simulink model "rigLoggerMultipacketRigH"  (R2012b)
settings: Solver=FixedStepDiscrete  StartTime=0.0  StopTime=10.0  FixedStep=0.001  RelTol=1e-3
values from neighbouring files (symbols this model uses):
  modelConstants = modelDefinedConstants()    [multipacketTestStart.m]
undefined symbols (not defined in the file or in its folder): macaddr
libraries: simulink x42, xpcethernetlib x29, xpcnetworkbufferlib x15, xpcutilitieslib x14, dspswit3 x14, dspmtrx3 x14, Lib_FileLoggerMultipacket x1
(part 1 of 6)
settings Model: BufferReuse=off  Creator=gilja  LastModifiedBy=NPTL
settings SolverCC: EnableConcurrentExecution=on  ConcurrentTasks=on
settings DataIOCC: SaveOutput=off  SignalLogging=off  SaveTime=off
settings OptimizationCC: InlineParams=on  InlineInvariantSignals=on  OptimizeBlockIOStorage=off  BufferReuse=off  ExpressionFolding=off  LocalBlockOutputs=off  SimCompilerOptimization=On
settings HardwareCC: ProdIntDivRoundTo=Zero  ProdEndianess=LittleEndian  ProdHWDeviceType=Generic->32-bit x86 compatible
settings ModelReferenceCC: ModelReferenceNumInstancesAllowed=Single  ModelReferenceMinAlgLoopOccurrences=on
settings RTWCC: SystemTargetFile=xpctarget.tlc  TemplateMakefile=xpc_default_tmf  Description=xPC Target  ProcessScript=xpctarget_make_rtw_hook  RTWCompilerOptimization=On
settings CodeAppCC: MaxIdLength=62
settings xpcTargetCC: TargetFcnLib=ansi_tfl_table_tmw.mat  CodeReplacementLibrary=XPC_BLAS  ParMdlRefBuildCompliant=on  ConcurrentExecutionCompliant=on  CombineSignalStateStructs=off  GRTInterface=on  RL32LogTETModifier=off  xPCTaskExecutionProfile=off  xPCRL32EventNumber=5000  xPCisDownloadable=off  xPCLoadParamSetFile=off  xPCConcurrentTasks=off  xPCEnableSFAnimation=off

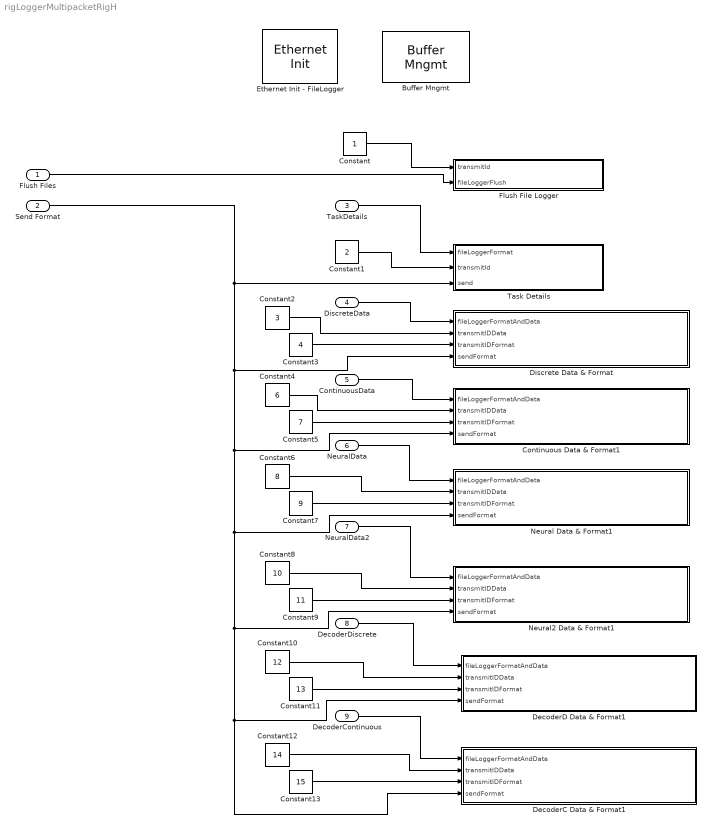
== system rigLoggerMultipacketRigH ==
  Flush Files : Inport  OutDataTypeStr=boolean
  Send Format : Inport  Port=2  OutDataTypeStr=boolean
  TaskDetails : Inport  Port=3  OutDataTypeStr=Bus: fileLoggerFormat
  DiscreteData : Inport  Port=4  OutDataTypeStr=Bus: fileLoggerFormatAndData
  ContinuousData : Inport  Port=5  OutDataTypeStr=Bus: fileLoggerFormatAndData
  NeuralData : Inport  Port=6  OutDataTypeStr=Bus: fileLoggerFormatAndData
  NeuralData2 : Inport  Port=7  OutDataTypeStr=Bus: fileLoggerFormatAndData
  DecoderDiscrete : Inport  Port=8  OutDataTypeStr=Bus: fileLoggerFormatAndData
  DecoderContinuous : Inport  Port=9  OutDataTypeStr=Bus: fileLoggerFormatAndData
  "Buffer Mngmt " : xpcnetworkbufferlib/Buffer Mngmt   Priority=-1  SampleTime=-1  PoolSizes=[8196 512 4096 65535]  ShowTune=on
  Constant : Constant  OutDataTypeStr=uint8
  Constant1 : Constant  Value=2  OutDataTypeStr=uint8
  Constant10 : Constant  Value=12  OutDataTypeStr=uint8
  Constant11 : Constant  Value=13  OutDataTypeStr=uint8
  Constant12 : Constant  Value=14  OutDataTypeStr=uint8
  Constant13 : Constant  Value=15  OutDataTypeStr=uint8
  Constant2 : Constant  Value=3  OutDataTypeStr=uint8
  Constant3 : Constant  Value=4  OutDataTypeStr=uint8
  Constant4 : Constant  Value=6  OutDataTypeStr=uint8
  Constant5 : Constant  Value=7  OutDataTypeStr=uint8
  Constant6 : Constant  Value=8  OutDataTypeStr=uint8
  Constant7 : Constant  Value=9  OutDataTypeStr=uint8
  Constant8 : Constant  Value=10  OutDataTypeStr=uint8
  Constant9 : Constant  Value=11  OutDataTypeStr=uint8
  Continuous Data & Format1 : Subsystem
  DecoderC Data & Format1 : Subsystem
  DecoderD Data & Format1 : Subsystem
  Discrete Data & Format : Subsystem
  Ethernet Init - FileLogger : xpcethernetlib/Ethernet Init   Priority=-1  ID=2  Driver=Intel Gigabit  Bus=6  Slot=0  SampleTime=-1  AddressSource=Specify  MAC=macaddr('00:00:00:00:00:00')  TxSA=off  RxPromiscuous=off  Multicast={}  RxBad=off  RxShort=off  MaxMTU=1518  TxThreshold=10  TxBuffers=128  RxBuffers=8  ShowTune=on  NumRxBlks=1
  Flush File Logger : Subsystem
  Neural Data & Format1 : Subsystem
  Neural2 Data & Format1 : Subsystem
  Task Details : Subsystem
  wires:
  Flush Files/1 -> Flush File Logger/2(fileLoggerFlush)
  TaskDetails/1 -> Task Details/1(fileLoggerFormat)
  ContinuousData/1 -> Continuous Data & Format1/1(fileLoggerFormatAndData)
  DiscreteData/1 -> Discrete Data & Format/1(fileLoggerFormatAndData)
  NeuralData/1 -> Neural Data & Format1/1(fileLoggerFormatAndData)
  DecoderDiscrete/1 -> DecoderD Data & Format1/1(fileLoggerFormatAndData)
  DecoderContinuous/1 -> DecoderC Data & Format1/1(fileLoggerFormatAndData)
  Send Format/1 -> Task Details/3(send), Discrete Data & Format/4(sendFormat), Continuous Data & Format1/4(sendFormat), Neural Data & Format1/4(sendFormat), Neural2 Data & Format1/4(sendFormat), DecoderD Data & Format1/4(sendFormat), DecoderC Data & Format1/4(sendFormat)
  NeuralData2/1 -> Neural2 Data & Format1/1(fileLoggerFormatAndData)
  Constant/1 -> Flush File Logger/1(transmitId)
  Constant1/1 -> Task Details/2(transmitId)
  Constant2/1 -> Discrete Data & Format/2(transmitIDData)
  Constant3/1 -> Discrete Data & Format/3(transmitIDFormat)
  Constant4/1 -> Continuous Data & Format1/2(transmitIDData)
  Constant5/1 -> Continuous Data & Format1/3(transmitIDFormat)
  Constant6/1 -> Neural Data & Format1/2(transmitIDData)
  Constant7/1 -> Neural Data & Format1/3(transmitIDFormat)
  Constant8/1 -> Neural2 Data & Format1/2(transmitIDData)
  Constant9/1 -> Neural2 Data & Format1/3(transmitIDFormat)
  Constant10/1 -> DecoderD Data & Format1/2(transmitIDData)
  Constant11/1 -> DecoderD Data & Format1/3(transmitIDFormat)
  Constant12/1 -> DecoderC Data & Format1/2(transmitIDData)
  Constant13/1 -> DecoderC Data & Format1/3(transmitIDFormat)

== system rigLoggerMultipacketRigH/Continuous Data & Format1 ==
  fileLoggerFormatAndData : Inport  OutDataTypeStr=Bus: fileLoggerFormatAndData
  transmitIDData : Inport  Port=2  OutDataTypeStr=uint8
  transmitIDFormat : Inport  Port=3  OutDataTypeStr=uint8
  sendFormat : Inport  Port=4  OutDataTypeStr=boolean
  Bus Selector2 : BusSelector  OutputSignals=data,format
  File Logger Data : Subsystem
  File Logger Format : Subsystem
  wires:
  transmitIDFormat/1 -> File Logger Format/2(transmitId)
  transmitIDData/1 -> File Logger Data/2(transmitId)
  sendFormat/1 -> File Logger Format/3(send)
  Bus Selector2/2 -> File Logger Format/1(fileLoggerFormat)  "<format>"
  Bus Selector2/1 -> File Logger Data/1(fileLoggerData)  "<data>"
  fileLoggerFormatAndData/1 -> Bus Selector2/1

== system rigLoggerMultipacketRigH/DecoderC Data & Format1 ==
  fileLoggerFormatAndData : Inport  OutDataTypeStr=Bus: fileLoggerFormatAndData
  transmitIDData : Inport  Port=2  OutDataTypeStr=uint8
  transmitIDFormat : Inport  Port=3  OutDataTypeStr=uint8
  sendFormat : Inport  Port=4  OutDataTypeStr=boolean
  Bus Selector2 : BusSelector  OutputSignals=data,format
  File Logger Data : Subsystem
  File Logger Format : Subsystem
  wires:
  transmitIDFormat/1 -> File Logger Format/2(transmitId)
  transmitIDData/1 -> File Logger Data/2(transmitId)
  sendFormat/1 -> File Logger Format/3(send)
  Bus Selector2/2 -> File Logger Format/1(fileLoggerFormat)  "<format>"
  Bus Selector2/1 -> File Logger Data/1(fileLoggerData)  "<data>"
  fileLoggerFormatAndData/1 -> Bus Selector2/1

== system rigLoggerMultipacketRigH/DecoderD Data & Format1 ==
  fileLoggerFormatAndData : Inport  OutDataTypeStr=Bus: fileLoggerFormatAndData
  transmitIDData : Inport  Port=2  OutDataTypeStr=uint8
  transmitIDFormat : Inport  Port=3  OutDataTypeStr=uint8
  sendFormat : Inport  Port=4  OutDataTypeStr=boolean
  Bus Selector2 : BusSelector  OutputSignals=data,format
  File Logger Data : Subsystem
  File Logger Format : Subsystem
  wires:
  transmitIDFormat/1 -> File Logger Format/2(transmitId)
  transmitIDData/1 -> File Logger Data/2(transmitId)
  sendFormat/1 -> File Logger Format/3(send)
  Bus Selector2/2 -> File Logger Format/1(fileLoggerFormat)  "<format>"
  Bus Selector2/1 -> File Logger Data/1(fileLoggerData)  "<data>"
  fileLoggerFormatAndData/1 -> Bus Selector2/1

== system rigLoggerMultipacketRigH/Discrete Data & Format ==
  fileLoggerFormatAndData : Inport  OutDataTypeStr=Bus: fileLoggerFormatAndData
  transmitIDData : Inport  Port=2  OutDataTypeStr=uint8
  transmitIDFormat : Inport  Port=3  OutDataTypeStr=uint8
  sendFormat : Inport  Port=4  OutDataTypeStr=boolean
  Bus Selector2 : BusSelector  OutputSignals=data,format
  File Logger Data : Subsystem
  File Logger Format : Subsystem
  wires:
  transmitIDFormat/1 -> File Logger Format/2(transmitId)
  transmitIDData/1 -> File Logger Data/2(transmitId)
  sendFormat/1 -> File Logger Format/3(send)
  Bus Selector2/2 -> File Logger Format/1(fileLoggerFormat)  "<format>"
  Bus Selector2/1 -> File Logger Data/1(fileLoggerData)  "<data>"
  fileLoggerFormatAndData/1 -> Bus Selector2/1

== system rigLoggerMultipacketRigH/Flush File Logger ==
  transmitId : Inport  OutDataTypeStr=uint8
  fileLoggerFlush : Inport  Port=2  OutDataTypeStr=boolean
  Constant1 : Constant  Value=0  OutDataTypeStr=boolean
  Constant4 : Constant  Value=0  OutDataTypeStr=uint8
  Constant7 : Constant  OutDataTypeStr=uint16
  Subsystem : Subsystem
  test.dat4 : Constant  Value=[uint8('flush') 0]  OutDataTypeStr=uint8
  wires:
  transmitId/1 -> Subsystem/5(transmitID)
  test.dat4/1 -> Subsystem/2(FileName)
  Constant1/1 -> Subsystem/1(Packet Type)
  Constant7/1 -> Subsystem/4(DataLen)
  fileLoggerFlush/1 -> Subsystem/6(Enable)
  Constant4/1 -> Subsystem/3(Data)

== system rigLoggerMultipacketRigH/Neural Data & Format1 ==
  fileLoggerFormatAndData : Inport  OutDataTypeStr=Bus: fileLoggerFormatAndData
  transmitIDData : Inport  Port=2  OutDataTypeStr=uint8
  transmitIDFormat : Inport  Port=3  OutDataTypeStr=uint8
  sendFormat : Inport  Port=4  OutDataTypeStr=boolean
  Bus Selector2 : BusSelector  OutputSignals=data,format
  File Logger Data : Subsystem
  File Logger Format : Subsystem
  wires:
  transmitIDFormat/1 -> File Logger Format/2(transmitId)
  transmitIDData/1 -> File Logger Data/2(transmitId)
  sendFormat/1 -> File Logger Format/3(send)
  Bus Selector2/2 -> File Logger Format/1(fileLoggerFormat)  "<format>"
  Bus Selector2/1 -> File Logger Data/1(fileLoggerData)  "<data>"
  fileLoggerFormatAndData/1 -> Bus Selector2/1

== system rigLoggerMultipacketRigH/Neural2 Data & Format1 ==
  fileLoggerFormatAndData : Inport  OutDataTypeStr=Bus: fileLoggerFormatAndData
  transmitIDData : Inport  Port=2  OutDataTypeStr=uint8
  transmitIDFormat : Inport  Port=3  OutDataTypeStr=uint8
  sendFormat : Inport  Port=4  OutDataTypeStr=boolean
  Bus Selector2 : BusSelector  OutputSignals=data,format
  File Logger Data : Subsystem
  File Logger Format : Subsystem
  wires:
  transmitIDFormat/1 -> File Logger Format/2(transmitId)
  transmitIDData/1 -> File Logger Data/2(transmitId)
  sendFormat/1 -> File Logger Format/3(send)
  Bus Selector2/2 -> File Logger Format/1(fileLoggerFormat)  "<format>"
  Bus Selector2/1 -> File Logger Data/1(fileLoggerData)  "<data>"
  fileLoggerFormatAndData/1 -> Bus Selector2/1

== system rigLoggerMultipacketRigH/Task Details ==
  fileLoggerFormat : Inport  OutDataTypeStr=Bus: fileLoggerFormat
  transmitId : Inport  Port=2  OutDataTypeStr=uint8
  send : Inport  Port=3  OutDataTypeStr=boolean
  Bus Selector2 : BusSelector  OutputSignals=fileName,format,formatLen
  Constant : Constant  OutDataTypeStr=boolean
  File Logger Multipacket : Subsystem
  wires:
  transmitId/1 -> File Logger Multipacket/5(transmitID)
  send/1 -> File Logger Multipacket/6(Enable)
  Bus Selector2/1 -> File Logger Multipacket/2(FileName)  "<fileName>"
  Bus Selector2/2 -> File Logger Multipacket/3(Data)  "<format>"
  Bus Selector2/3 -> File Logger Multipacket/4(DataLen)  "<formatLen>"
  Constant/1 -> File Logger Multipacket/1(Packet Type)
  fileLoggerFormat/1 -> Bus Selector2/1

== system rigLoggerMultipacketRigH/Continuous Data & Format1/File Logger Data ==
  fileLoggerData : Inport  OutDataTypeStr=Bus: fileLoggerData
  transmitId : Inport  Port=2  OutDataTypeStr=uint8
  Bus Selector2 : BusSelector  OutputSignals=send,fileName,data,dataLen
  Constant : Constant  OutDataTypeStr=boolean
  File Logger Multipacket : Subsystem
  wires:
  transmitId/1 -> File Logger Multipacket/5(transmitID)
  Bus Selector2/2 -> File Logger Multipacket/2(FileName)  "<fileName>"
  Bus Selector2/3 -> File Logger Multipacket/3(Data)  "<data>"
  Bus Selector2/4 -> File Logger Multipacket/4(DataLen)  "<dataLen>"
  Bus Selector2/1 -> File Logger Multipacket/6(Enable)  "<send>"
  Constant/1 -> File Logger Multipacket/1(Packet Type)
  fileLoggerData/1 -> Bus Selector2/1

== system rigLoggerMultipacketRigH/Continuous Data & Format1/File Logger Format ==
  fileLoggerFormat : Inport  OutDataTypeStr=Bus: fileLoggerFormat
  transmitId : Inport  Port=2  OutDataTypeStr=uint8
  send : Inport  Port=3  OutDataTypeStr=boolean
  Bus Selector2 : BusSelector  OutputSignals=fileName,format,formatLen
  Constant : Constant  OutDataTypeStr=boolean
  File Logger Multipacket : Subsystem
  wires:
  transmitId/1 -> File Logger Multipacket/5(transmitID)
  send/1 -> File Logger Multipacket/6(Enable)
  Bus Selector2/1 -> File Logger Multipacket/2(FileName)  "<fileName>"
  Bus Selector2/2 -> File Logger Multipacket/3(Data)  "<format>"
  Bus Selector2/3 -> File Logger Multipacket/4(DataLen)  "<formatLen>"
  Constant/1 -> File Logger Multipacket/1(Packet Type)
  fileLoggerFormat/1 -> Bus Selector2/1

== system rigLoggerMultipacketRigH/DecoderC Data & Format1/File Logger Data ==
  fileLoggerData : Inport  OutDataTypeStr=Bus: fileLoggerData
  transmitId : Inport  Port=2  OutDataTypeStr=uint8
  Bus Selector2 : BusSelector  OutputSignals=send,fileName,data,dataLen
  Constant : Constant  OutDataTypeStr=boolean
  File Logger Multipacket : Subsystem
  wires:
  transmitId/1 -> File Logger Multipacket/5(transmitID)
  Bus Selector2/2 -> File Logger Multipacket/2(FileName)  "<fileName>"
  Bus Selector2/3 -> File Logger Multipacket/3(Data)  "<data>"
  Bus Selector2/4 -> File Logger Multipacket/4(DataLen)  "<dataLen>"
  Bus Selector2/1 -> File Logger Multipacket/6(Enable)  "<send>"
  Constant/1 -> File Logger Multipacket/1(Packet Type)
  fileLoggerData/1 -> Bus Selector2/1

== system rigLoggerMultipacketRigH/DecoderC Data & Format1/File Logger Format ==
  fileLoggerFormat : Inport  OutDataTypeStr=Bus: fileLoggerFormat
  transmitId : Inport  Port=2  OutDataTypeStr=uint8
  send : Inport  Port=3  OutDataTypeStr=boolean
  Bus Selector2 : BusSelector  OutputSignals=fileName,format,formatLen
  Constant : Constant  OutDataTypeStr=boolean
  File Logger Multipacket : Subsystem
  wires:
  transmitId/1 -> File Logger Multipacket/5(transmitID)
  send/1 -> File Logger Multipacket/6(Enable)
  Bus Selector2/1 -> File Logger Multipacket/2(FileName)  "<fileName>"
  Bus Selector2/2 -> File Logger Multipacket/3(Data)  "<format>"
  Bus Selector2/3 -> File Logger Multipacket/4(DataLen)  "<formatLen>"
  Constant/1 -> File Logger Multipacket/1(Packet Type)
  fileLoggerFormat/1 -> Bus Selector2/1

== system rigLoggerMultipacketRigH/DecoderD Data & Format1/File Logger Data ==
  fileLoggerData : Inport  OutDataTypeStr=Bus: fileLoggerData
  transmitId : Inport  Port=2  OutDataTypeStr=uint8
  Bus Selector2 : BusSelector  OutputSignals=send,fileName,data,dataLen
  Constant : Constant  OutDataTypeStr=boolean
  File Logger Multipacket : Subsystem
  wires:
  transmitId/1 -> File Logger Multipacket/5(transmitID)
  Bus Selector2/2 -> File Logger Multipacket/2(FileName)  "<fileName>"
  Bus Selector2/3 -> File Logger Multipacket/3(Data)  "<data>"
  Bus Selector2/4 -> File Logger Multipacket/4(DataLen)  "<dataLen>"
  Bus Selector2/1 -> File Logger Multipacket/6(Enable)  "<send>"
  Constant/1 -> File Logger Multipacket/1(Packet Type)
  fileLoggerData/1 -> Bus Selector2/1

== system rigLoggerMultipacketRigH/DecoderD Data & Format1/File Logger Format ==
  fileLoggerFormat : Inport  OutDataTypeStr=Bus: fileLoggerFormat
  transmitId : Inport  Port=2  OutDataTypeStr=uint8
  send : Inport  Port=3  OutDataTypeStr=boolean
  Bus Selector2 : BusSelector  OutputSignals=fileName,format,formatLen
  Constant : Constant  OutDataTypeStr=boolean
  File Logger Multipacket : Subsystem
  wires:
  transmitId/1 -> File Logger Multipacket/5(transmitID)
  send/1 -> File Logger Multipacket/6(Enable)
  Bus Selector2/1 -> File Logger Multipacket/2(FileName)  "<fileName>"
  Bus Selector2/2 -> File Logger Multipacket/3(Data)  "<format>"
  Bus Selector2/3 -> File Logger Multipacket/4(DataLen)  "<formatLen>"
  Constant/1 -> File Logger Multipacket/1(Packet Type)
  fileLoggerFormat/1 -> Bus Selector2/1

== system rigLoggerMultipacketRigH/Discrete Data & Format/File Logger Data ==
  fileLoggerData : Inport  OutDataTypeStr=Bus: fileLoggerData
  transmitId : Inport  Port=2  OutDataTypeStr=uint8
  Bus Selector2 : BusSelector  OutputSignals=send,fileName,data,dataLen
  Constant : Constant  OutDataTypeStr=boolean
  File Logger Multipacket : Subsystem
  wires:
  transmitId/1 -> File Logger Multipacket/5(transmitID)
  Bus Selector2/2 -> File Logger Multipacket/2(FileName)  "<fileName>"
  Bus Selector2/3 -> File Logger Multipacket/3(Data)  "<data>"
  Bus Selector2/4 -> File Logger Multipacket/4(DataLen)  "<dataLen>"
  Bus Selector2/1 -> File Logger Multipacket/6(Enable)  "<send>"
  Constant/1 -> File Logger Multipacket/1(Packet Type)
  fileLoggerData/1 -> Bus Selector2/1

== system rigLoggerMultipacketRigH/Discrete Data & Format/File Logger Format ==
  fileLoggerFormat : Inport  OutDataTypeStr=Bus: fileLoggerFormat
  transmitId : Inport  Port=2  OutDataTypeStr=uint8
  send : Inport  Port=3  OutDataTypeStr=boolean
  Bus Selector2 : BusSelector  OutputSignals=fileName,format,formatLen
  Constant : Constant  OutDataTypeStr=boolean
  File Logger Multipacket : Subsystem
  wires:
  transmitId/1 -> File Logger Multipacket/5(transmitID)
  send/1 -> File Logger Multipacket/6(Enable)
  Bus Selector2/1 -> File Logger Multipacket/2(FileName)  "<fileName>"
  Bus Selector2/2 -> File Logger Multipacket/3(Data)  "<format>"
  Bus Selector2/3 -> File Logger Multipacket/4(DataLen)  "<formatLen>"
  Constant/1 -> File Logger Multipacket/1(Packet Type)
  fileLoggerFormat/1 -> Bus Selector2/1

== system rigLoggerMultipacketRigH/Flush File Logger/Subsystem ==
  Packet Type : Inport
  FileName : Inport  Port=2
  Data : Inport  Port=3
  DataLen : Inport  Port=4
  transmitID : Inport  Port=5
  Enable : Inport  Port=6
  File Logger Wrapper : Subsystem
  MATLAB Function1 : Lib_FileLoggerMultipacket/File Logger Multipacket/MATLAB Function1
  Send Multipacket UDP : Subsystem  mask(Send Multipacket UDP Block){destMac=macaddr('ff:ff:ff:ff:ff:ff'), ID=2, prependHeader=off}
      mask prompts: destMac "Destination MAC:"; ID "Ethernet Device ID:"; prependHeader "Prepend 4-byte Header (uint16 length, uint16 checksum)"
      mask help: Splits a UDP packet into multiple pieces to be reassembled at the receiver
      mask TypeOptions ID: Ethernet Tx /ID
      mask Display:
      | disp([ 'Ethernet Tx ' num2str(ID)]);
      | port_label('input', 1, 'sourceIp');
      | port_label('input', 2, 'destIp');
      | port_label('input', 3, 'sourcePort');
      | port_label('input', 4, 'destPort');
      | port_label('input', 5, 'data (uint8)');
      | port_label('input', 6, 'transmitId (uint8)');
      | port_label('Enable','Enable')
  dIP : Constant  Value=modelConstants.filelogging.ip  OutDataTypeStr=uint8
  dPort : Constant  Value=modelConstants.filelogging.RECV_PORT  OutDataTypeStr=uint16
  sIP : Constant  Value=modelConstants.filelogging.xPCip  OutDataTypeStr=uint8
  sPort : Constant  Value=modelConstants.filelogging.SRC_PORT  OutDataTypeStr=uint16
  wires:
  FileName/1 -> MATLAB Function1/1
  Packet Type/1 -> File Logger Wrapper/1(Packet Type)
  MATLAB Function1/1 -> File Logger Wrapper/2(FileName)
  File Logger Wrapper/2(UDP Size) -> ?
  DataLen/1 -> File Logger Wrapper/4(FrameSize)
  Data/1 -> File Logger Wrapper/3(Frame)
  Enable/1 -> Send Multipacket UDP/Enable
  dPort/1 -> Send Multipacket UDP/4(destPort)
  sPort/1 -> Send Multipacket UDP/3(sourcePort)
  dIP/1 -> Send Multipacket UDP/2(destIP)
  sIP/1 -> Send Multipacket UDP/1(sourceIP)
  File Logger Wrapper/1(UDP Data) -> Send Multipacket UDP/5(Data)
  transmitID/1 -> Send Multipacket UDP/6(transmitId)

== system rigLoggerMultipacketRigH/Neural Data & Format1/File Logger Data ==
  fileLoggerData : Inport  OutDataTypeStr=Bus: fileLoggerData
  transmitId : Inport  Port=2  OutDataTypeStr=uint8
  Bus Selector2 : BusSelector  OutputSignals=send,fileName,data,dataLen
  Constant : Constant  OutDataTypeStr=boolean
  File Logger Multipacket : Subsystem
  wires:
  transmitId/1 -> File Logger Multipacket/5(transmitID)
  Bus Selector2/2 -> File Logger Multipacket/2(FileName)  "<fileName>"
  Bus Selector2/3 -> File Logger Multipacket/3(Data)  "<data>"
  Bus Selector2/4 -> File Logger Multipacket/4(DataLen)  "<dataLen>"
  Bus Selector2/1 -> File Logger Multipacket/6(Enable)  "<send>"
  Constant/1 -> File Logger Multipacket/1(Packet Type)
  fileLoggerData/1 -> Bus Selector2/1

== system rigLoggerMultipacketRigH/Neural Data & Format1/File Logger Format ==
  fileLoggerFormat : Inport  OutDataTypeStr=Bus: fileLoggerFormat
  transmitId : Inport  Port=2  OutDataTypeStr=uint8
  send : Inport  Port=3  OutDataTypeStr=boolean
  Bus Selector2 : BusSelector  OutputSignals=fileName,format,formatLen
  Constant : Constant  OutDataTypeStr=boolean
  File Logger Multipacket : Subsystem
  wires:
  transmitId/1 -> File Logger Multipacket/5(transmitID)
  send/1 -> File Logger Multipacket/6(Enable)
  Bus Selector2/1 -> File Logger Multipacket/2(FileName)  "<fileName>"
  Bus Selector2/2 -> File Logger Multipacket/3(Data)  "<format>"
  Bus Selector2/3 -> File Logger Multipacket/4(DataLen)  "<formatLen>"
  Constant/1 -> File Logger Multipacket/1(Packet Type)
  fileLoggerFormat/1 -> Bus Selector2/1

== system rigLoggerMultipacketRigH/Neural2 Data & Format1/File Logger Data ==
  fileLoggerData : Inport  OutDataTypeStr=Bus: fileLoggerData
  transmitId : Inport  Port=2  OutDataTypeStr=uint8
  Bus Selector2 : BusSelector  OutputSignals=send,fileName,data,dataLen
  Constant : Constant  OutDataTypeStr=boolean
  File Logger Multipacket : Subsystem
  wires:
  transmitId/1 -> File Logger Multipacket/5(transmitID)
  Bus Selector2/2 -> File Logger Multipacket/2(FileName)  "<fileName>"
  Bus Selector2/3 -> File Logger Multipacket/3(Data)  "<data>"
  Bus Selector2/4 -> File Logger Multipacket/4(DataLen)  "<dataLen>"
  Bus Selector2/1 -> File Logger Multipacket/6(Enable)  "<send>"
  Constant/1 -> File Logger Multipacket/1(Packet Type)
  fileLoggerData/1 -> Bus Selector2/1

== system rigLoggerMultipacketRigH/Neural2 Data & Format1/File Logger Format ==
  fileLoggerFormat : Inport  OutDataTypeStr=Bus: fileLoggerFormat
  transmitId : Inport  Port=2  OutDataTypeStr=uint8
  send : Inport  Port=3  OutDataTypeStr=boolean
  Bus Selector2 : BusSelector  OutputSignals=fileName,format,formatLen
  Constant : Constant  OutDataTypeStr=boolean
  File Logger Multipacket : Subsystem
  wires:
  transmitId/1 -> File Logger Multipacket/5(transmitID)
  send/1 -> File Logger Multipacket/6(Enable)
  Bus Selector2/1 -> File Logger Multipacket/2(FileName)  "<fileName>"
  Bus Selector2/2 -> File Logger Multipacket/3(Data)  "<format>"
  Bus Selector2/3 -> File Logger Multipacket/4(DataLen)  "<formatLen>"
  Constant/1 -> File Logger Multipacket/1(Packet Type)
  fileLoggerFormat/1 -> Bus Selector2/1

== system rigLoggerMultipacketRigH/Task Details/File Logger Multipacket ==
  Packet Type : Inport
  FileName : Inport  Port=2
  Data : Inport  Port=3
  DataLen : Inport  Port=4
  transmitID : Inport  Port=5
  Enable : Inport  Port=6
  File Logger Wrapper : Subsystem
  MATLAB Function1 : MATLAB Function  TreatAsAtomicUnit=on
  Send Multipacket UDP : Subsystem  mask(Send Multipacket UDP Block){destMac=macaddr('ff:ff:ff:ff:ff:ff'), ID=2, prependHeader=off}
      mask prompts: destMac "Destination MAC:"; ID "Ethernet Device ID:"; prependHeader "Prepend 4-byte Header (uint16 length, uint16 checksum)"
      mask help: Splits a UDP packet into multiple pieces to be reassembled at the receiver
      mask TypeOptions ID: Ethernet Tx /ID
      mask Display:
      | disp([ 'Ethernet Tx ' num2str(ID)]);
      | port_label('input', 1, 'sourceIp');
      | port_label('input', 2, 'destIp');
      | port_label('input', 3, 'sourcePort');
      | port_label('input', 4, 'destPort');
      | port_label('input', 5, 'data (uint8)');
      | port_label('input', 6, 'transmitId (uint8)');
      | port_label('Enable','Enable')
  dIP : Constant  Value=modelConstants.filelogging.ip  OutDataTypeStr=uint8
  dPort : Constant  Value=modelConstants.filelogging.RECV_PORT  OutDataTypeStr=uint16
  sIP : Constant  Value=modelConstants.filelogging.xPCip  OutDataTypeStr=uint8
  sPort : Constant  Value=modelConstants.filelogging.SRC_PORT  OutDataTypeStr=uint16
  wires:
  transmitID/1 -> Send Multipacket UDP/6(transmitId)
  File Logger Wrapper/1(UDP Data) -> Send Multipacket UDP/5(Data)
  sIP/1 -> Send Multipacket UDP/1(sourceIP)
  dIP/1 -> Send Multipacket UDP/2(destIP)
  sPort/1 -> Send Multipacket UDP/3(sourcePort)
  dPort/1 -> Send Multipacket UDP/4(destPort)
  Enable/1 -> Send Multipacket UDP/Enable
  Data/1 -> File Logger Wrapper/3(Frame)
  DataLen/1 -> File Logger Wrapper/4(FrameSize)
  File Logger Wrapper/2(UDP Size) -> ?
  MATLAB Function1/1(y) -> File Logger Wrapper/2(FileName)
  Packet Type/1 -> File Logger Wrapper/1(Packet Type)
  FileName/1 -> MATLAB Function1/1(u)

== system rigLoggerMultipacketRigH/Continuous Data & Format1/File Logger Data/File Logger Multipacket ==
  Packet Type : Inport
  FileName : Inport  Port=2
  Data : Inport  Port=3
  DataLen : Inport  Port=4
  transmitID : Inport  Port=5
  Enable : Inport  Port=6
  File Logger Wrapper : Subsystem
  MATLAB Function1 : MATLAB Function  TreatAsAtomicUnit=on
  MATLAB Function2 : MATLAB Function  TreatAsAtomicUnit=on
  MATLAB Function3 : MATLAB Function  TreatAsAtomicUnit=on
  Send Multipacket UDP : Subsystem  mask(Send Multipacket UDP Block){destMac=macaddr('ff:ff:ff:ff:ff:ff'), ID=2, prependHeader=off}
      mask prompts: destMac "Destination MAC:"; ID "Ethernet Device ID:"; prependHeader "Prepend 4-byte Header (uint16 length, uint16 checksum)"
      mask help: Splits a UDP packet into multiple pieces to be reassembled at the receiver
      mask TypeOptions ID: Ethernet Tx /ID
      mask Display:
      | disp([ 'Ethernet Tx ' num2str(ID)]);
      | port_label('input', 1, 'sourceIp');
      | port_label('input', 2, 'destIp');
      | port_label('input', 3, 'sourcePort');
      | port_label('input', 4, 'destPort');
      | port_label('input', 5, 'data (uint8)');
      | port_label('input', 6, 'transmitId (uint8)');
      | port_label('Enable','Enable')
  dIP : Constant  Value=modelConstants.filelogging.ip  OutDataTypeStr=uint8
  dPort : Constant  Value=modelConstants.filelogging.RECV_PORT  OutDataTypeStr=uint16
  sIP : Constant  Value=modelConstants.filelogging.xPCip  OutDataTypeStr=uint8
  sPort : Constant  Value=modelConstants.filelogging.SRC_PORT  OutDataTypeStr=uint16
  wires:
  transmitID/1 -> Send Multipacket UDP/6(transmitId)
  File Logger Wrapper/1(UDP Data) -> Send Multipacket UDP/5(Data)
  sIP/1 -> Send Multipacket UDP/1(sourceIP)
  dIP/1 -> Send Multipacket UDP/2(destIP)
  sPort/1 -> Send Multipacket UDP/3(sourcePort)
  dPort/1 -> Send Multipacket UDP/4(destPort)
  Enable/1 -> Send Multipacket UDP/Enable
  File Logger Wrapper/2(UDP Size) -> ?
  MATLAB Function1/1(y) -> File Logger Wrapper/2(FileName)
  Packet Type/1 -> File Logger Wrapper/1(Packet Type)
  FileName/1 -> MATLAB Function1/1(u)
  MATLAB Function2/1(y) -> File Logger Wrapper/3(Frame)
  Data/1 -> MATLAB Function2/1(u)
  DataLen/1 -> MATLAB Function3/1(u)
  MATLAB Function3/1(y) -> File Logger Wrapper/4(FrameSize)

== system rigLoggerMultipacketRigH/Continuous Data & Format1/File Logger Format/File Logger Multipacket ==
  Packet Type : Inport
  FileName : Inport  Port=2
  Data : Inport  Port=3
  DataLen : Inport  Port=4
  transmitID : Inport  Port=5
  Enable : Inport  Port=6
  File Logger Wrapper : Subsystem
  MATLAB Function1 : MATLAB Function  TreatAsAtomicUnit=on
  Send Multipacket UDP : Subsystem  mask(Send Multipacket UDP Block){destMac=macaddr('ff:ff:ff:ff:ff:ff'), ID=2, prependHeader=off}
      mask prompts: destMac "Destination MAC:"; ID "Ethernet Device ID:"; prependHeader "Prepend 4-byte Header (uint16 length, uint16 checksum)"
      mask help: Splits a UDP packet into multiple pieces to be reassembled at the receiver
      mask TypeOptions ID: Ethernet Tx /ID
      mask Display:
      | disp([ 'Ethernet Tx ' num2str(ID)]);
      | port_label('input', 1, 'sourceIp');
      | port_label('input', 2, 'destIp');
      | port_label('input', 3, 'sourcePort');
      | port_label('input', 4, 'destPort');
      | port_label('input', 5, 'data (uint8)');
      | port_label('input', 6, 'transmitId (uint8)');
      | port_label('Enable','Enable')
  dIP : Constant  Value=modelConstants.filelogging.ip  OutDataTypeStr=uint8
  dPort : Constant  Value=modelConstants.filelogging.RECV_PORT  OutDataTypeStr=uint16
  sIP : Constant  Value=modelConstants.filelogging.xPCip  OutDataTypeStr=uint8
  sPort : Constant  Value=modelConstants.filelogging.SRC_PORT  OutDataTypeStr=uint16
  wires:
  transmitID/1 -> Send Multipacket UDP/6(transmitId)
  File Logger Wrapper/1(UDP Data) -> Send Multipacket UDP/5(Data)
  sIP/1 -> Send Multipacket UDP/1(sourceIP)
  dIP/1 -> Send Multipacket UDP/2(destIP)
  sPort/1 -> Send Multipacket UDP/3(sourcePort)
  dPort/1 -> Send Multipacket UDP/4(destPort)
  Enable/1 -> Send Multipacket UDP/Enable
  Data/1 -> File Logger Wrapper/3(Frame)
  DataLen/1 -> File Logger Wrapper/4(FrameSize)
  File Logger Wrapper/2(UDP Size) -> ?
  MATLAB Function1/1(y) -> File Logger Wrapper/2(FileName)
  Packet Type/1 -> File Logger Wrapper/1(Packet Type)
  FileName/1 -> MATLAB Function1/1(u)

== system rigLoggerMultipacketRigH/DecoderC Data & Format1/File Logger Data/File Logger Multipacket ==
  Packet Type : Inport
  FileName : Inport  Port=2
  Data : Inport  Port=3
  DataLen : Inport  Port=4
  transmitID : Inport  Port=5
  Enable : Inport  Port=6
  File Logger Wrapper : Subsystem
  MATLAB Function1 : MATLAB Function  TreatAsAtomicUnit=on
  Send Multipacket UDP : Subsystem  mask(Send Multipacket UDP Block){destMac=macaddr('ff:ff:ff:ff:ff:ff'), ID=2, prependHeader=off}
      mask prompts: destMac "Destination MAC:"; ID "Ethernet Device ID:"; prependHeader "Prepend 4-byte Header (uint16 length, uint16 checksum)"
      mask help: Splits a UDP packet into multiple pieces to be reassembled at the receiver
      mask TypeOptions ID: Ethernet Tx /ID
      mask Display:
      | disp([ 'Ethernet Tx ' num2str(ID)]);
      | port_label('input', 1, 'sourceIp');
      | port_label('input', 2, 'destIp');
      | port_label('input', 3, 'sourcePort');
      | port_label('input', 4, 'destPort');
      | port_label('input', 5, 'data (uint8)');
      | port_label('input', 6, 'transmitId (uint8)');
      | port_label('Enable','Enable')
  dIP : Constant  Value=modelConstants.filelogging.ip  OutDataTypeStr=uint8
  dPort : Constant  Value=modelConstants.filelogging.RECV_PORT  OutDataTypeStr=uint16
  sIP : Constant  Value=modelConstants.filelogging.xPCip  OutDataTypeStr=uint8
  sPort : Constant  Value=modelConstants.filelogging.SRC_PORT  OutDataTypeStr=uint16
  wires:
  transmitID/1 -> Send Multipacket UDP/6(transmitId)
  File Logger Wrapper/1(UDP Data) -> Send Multipacket UDP/5(Data)
  sIP/1 -> Send Multipacket UDP/1(sourceIP)
  dIP/1 -> Send Multipacket UDP/2(destIP)
  sPort/1 -> Send Multipacket UDP/3(sourcePort)
  dPort/1 -> Send Multipacket UDP/4(destPort)
  Enable/1 -> Send Multipacket UDP/Enable
  Data/1 -> File Logger Wrapper/3(Frame)
  DataLen/1 -> File Logger Wrapper/4(FrameSize)
  File Logger Wrapper/2(UDP Size) -> ?
  MATLAB Function1/1(y) -> File Logger Wrapper/2(FileName)
  Packet Type/1 -> File Logger Wrapper/1(Packet Type)
  FileName/1 -> MATLAB Function1/1(u)

== system rigLoggerMultipacketRigH/DecoderC Data & Format1/File Logger Format/File Logger Multipacket ==
  Packet Type : Inport
  FileName : Inport  Port=2
  Data : Inport  Port=3
  DataLen : Inport  Port=4
  transmitID : Inport  Port=5
  Enable : Inport  Port=6
  File Logger Wrapper : Subsystem
  MATLAB Function1 : MATLAB Function  TreatAsAtomicUnit=on
  Send Multipacket UDP : Subsystem  mask(Send Multipacket UDP Block){destMac=macaddr('ff:ff:ff:ff:ff:ff'), ID=2, prependHeader=off}
      mask prompts: destMac "Destination MAC:"; ID "Ethernet Device ID:"; prependHeader "Prepend 4-byte Header (uint16 length, uint16 checksum)"
      mask help: Splits a UDP packet into multiple pieces to be reassembled at the receiver
      mask TypeOptions ID: Ethernet Tx /ID
      mask Display:
      | disp([ 'Ethernet Tx ' num2str(ID)]);
      | port_label('input', 1, 'sourceIp');
      | port_label('input', 2, 'destIp');
      | port_label('input', 3, 'sourcePort');
      | port_label('input', 4, 'destPort');
      | port_label('input', 5, 'data (uint8)');
      | port_label('input', 6, 'transmitId (uint8)');
      | port_label('Enable','Enable')
  dIP : Constant  Value=modelConstants.filelogging.ip  OutDataTypeStr=uint8
  dPort : Constant  Value=modelConstants.filelogging.RECV_PORT  OutDataTypeStr=uint16
  sIP : Constant  Value=modelConstants.filelogging.xPCip  OutDataTypeStr=uint8
  sPort : Constant  Value=modelConstants.filelogging.SRC_PORT  OutDataTypeStr=uint16
  wires:
  transmitID/1 -> Send Multipacket UDP/6(transmitId)
  File Logger Wrapper/1(UDP Data) -> Send Multipacket UDP/5(Data)
  sIP/1 -> Send Multipacket UDP/1(sourceIP)
  dIP/1 -> Send Multipacket UDP/2(destIP)
  sPort/1 -> Send Multipacket UDP/3(sourcePort)
  dPort/1 -> Send Multipacket UDP/4(destPort)
  Enable/1 -> Send Multipacket UDP/Enable
  Data/1 -> File Logger Wrapper/3(Frame)
  DataLen/1 -> File Logger Wrapper/4(FrameSize)
  File Logger Wrapper/2(UDP Size) -> ?
  MATLAB Function1/1(y) -> File Logger Wrapper/2(FileName)
  Packet Type/1 -> File Logger Wrapper/1(Packet Type)
  FileName/1 -> MATLAB Function1/1(u)

== system rigLoggerMultipacketRigH/DecoderD Data & Format1/File Logger Data/File Logger Multipacket ==
  Packet Type : Inport
  FileName : Inport  Port=2
  Data : Inport  Port=3
  DataLen : Inport  Port=4
  transmitID : Inport  Port=5
  Enable : Inport  Port=6
  File Logger Wrapper : Subsystem
  MATLAB Function1 : MATLAB Function  TreatAsAtomicUnit=on
  Send Multipacket UDP : Subsystem  mask(Send Multipacket UDP Block){destMac=macaddr('ff:ff:ff:ff:ff:ff'), ID=2, prependHeader=off}
      mask prompts: destMac "Destination MAC:"; ID "Ethernet Device ID:"; prependHeader "Prepend 4-byte Header (uint16 length, uint16 checksum)"
      mask help: Splits a UDP packet into multiple pieces to be reassembled at the receiver
      mask TypeOptions ID: Ethernet Tx /ID
      mask Display:
      | disp([ 'Ethernet Tx ' num2str(ID)]);
      | port_label('input', 1, 'sourceIp');
      | port_label('input', 2, 'destIp');
      | port_label('input', 3, 'sourcePort');
      | port_label('input', 4, 'destPort');
      | port_label('input', 5, 'data (uint8)');
      | port_label('input', 6, 'transmitId (uint8)');
      | port_label('Enable','Enable')
  dIP : Constant  Value=modelConstants.filelogging.ip  OutDataTypeStr=uint8
  dPort : Constant  Value=modelConstants.filelogging.RECV_PORT  OutDataTypeStr=uint16
  sIP : Constant  Value=modelConstants.filelogging.xPCip  OutDataTypeStr=uint8
  sPort : Constant  Value=modelConstants.filelogging.SRC_PORT  OutDataTypeStr=uint16
  wires:
  transmitID/1 -> Send Multipacket UDP/6(transmitId)
  File Logger Wrapper/1(UDP Data) -> Send Multipacket UDP/5(Data)
  sIP/1 -> Send Multipacket UDP/1(sourceIP)
  dIP/1 -> Send Multipacket UDP/2(destIP)
  sPort/1 -> Send Multipacket UDP/3(sourcePort)
  dPort/1 -> Send Multipacket UDP/4(destPort)
  Enable/1 -> Send Multipacket UDP/Enable
  Data/1 -> File Logger Wrapper/3(Frame)
  DataLen/1 -> File Logger Wrapper/4(FrameSize)
  File Logger Wrapper/2(UDP Size) -> ?
  MATLAB Function1/1(y) -> File Logger Wrapper/2(FileName)
  Packet Type/1 -> File Logger Wrapper/1(Packet Type)
  FileName/1 -> MATLAB Function1/1(u)

== system rigLoggerMultipacketRigH/DecoderD Data & Format1/File Logger Format/File Logger Multipacket ==
  Packet Type : Inport
  FileName : Inport  Port=2
  Data : Inport  Port=3
  DataLen : Inport  Port=4
  transmitID : Inport  Port=5
  Enable : Inport  Port=6
  File Logger Wrapper : Subsystem
  MATLAB Function1 : MATLAB Function  TreatAsAtomicUnit=on
  Send Multipacket UDP : Subsystem  mask(Send Multipacket UDP Block){destMac=macaddr('ff:ff:ff:ff:ff:ff'), ID=2, prependHeader=off}
      mask prompts: destMac "Destination MAC:"; ID "Ethernet Device ID:"; prependHeader "Prepend 4-byte Header (uint16 length, uint16 checksum)"
      mask help: Splits a UDP packet into multiple pieces to be reassembled at the receiver
      mask TypeOptions ID: Ethernet Tx /ID
      mask Display:
      | disp([ 'Ethernet Tx ' num2str(ID)]);
      | port_label('input', 1, 'sourceIp');
      | port_label('input', 2, 'destIp');
      | port_label('input', 3, 'sourcePort');
      | port_label('input', 4, 'destPort');
      | port_label('input', 5, 'data (uint8)');
      | port_label('input', 6, 'transmitId (uint8)');
      | port_label('Enable','Enable')
  dIP : Constant  Value=modelConstants.filelogging.ip  OutDataTypeStr=uint8
  dPort : Constant  Value=modelConstants.filelogging.RECV_PORT  OutDataTypeStr=uint16
  sIP : Constant  Value=modelConstants.filelogging.xPCip  OutDataTypeStr=uint8
  sPort : Constant  Value=modelConstants.filelogging.SRC_PORT  OutDataTypeStr=uint16
  wires:
  transmitID/1 -> Send Multipacket UDP/6(transmitId)
  File Logger Wrapper/1(UDP Data) -> Send Multipacket UDP/5(Data)
  sIP/1 -> Send Multipacket UDP/1(sourceIP)
  dIP/1 -> Send Multipacket UDP/2(destIP)
  sPort/1 -> Send Multipacket UDP/3(sourcePort)
  dPort/1 -> Send Multipacket UDP/4(destPort)
  Enable/1 -> Send Multipacket UDP/Enable
  Data/1 -> File Logger Wrapper/3(Frame)
  DataLen/1 -> File Logger Wrapper/4(FrameSize)
  File Logger Wrapper/2(UDP Size) -> ?
  MATLAB Function1/1(y) -> File Logger Wrapper/2(FileName)
  Packet Type/1 -> File Logger Wrapper/1(Packet Type)
  FileName/1 -> MATLAB Function1/1(u)

== system rigLoggerMultipacketRigH/Discrete Data & Format/File Logger Data/File Logger Multipacket ==
  Packet Type : Inport
  FileName : Inport  Port=2
  Data : Inport  Port=3
  DataLen : Inport  Port=4
  transmitID : Inport  Port=5
  Enable : Inport  Port=6
  File Logger Wrapper : Subsystem
  MATLAB Function1 : MATLAB Function  TreatAsAtomicUnit=on
  Send Multipacket UDP : Subsystem  mask(Send Multipacket UDP Block){destMac=macaddr('ff:ff:ff:ff:ff:ff'), ID=2, prependHeader=off}
      mask prompts: destMac "Destination MAC:"; ID "Ethernet Device ID:"; prependHeader "Prepend 4-byte Header (uint16 length, uint16 checksum)"
      mask help: Splits a UDP packet into multiple pieces to be reassembled at the receiver
      mask TypeOptions ID: Ethernet Tx /ID
      mask Display:
      | disp([ 'Ethernet Tx ' num2str(ID)]);
      | port_label('input', 1, 'sourceIp');
      | port_label('input', 2, 'destIp');
      | port_label('input', 3, 'sourcePort');
      | port_label('input', 4, 'destPort');
      | port_label('input', 5, 'data (uint8)');
      | port_label('input', 6, 'transmitId (uint8)');
      | port_label('Enable','Enable')
  dIP : Constant  Value=modelConstants.filelogging.ip  OutDataTypeStr=uint8
  dPort : Constant  Value=modelConstants.filelogging.RECV_PORT  OutDataTypeStr=uint16
  sIP : Constant  Value=modelConstants.filelogging.xPCip  OutDataTypeStr=uint8
  sPort : Constant  Value=modelConstants.filelogging.SRC_PORT  OutDataTypeStr=uint16
  wires:
  transmitID/1 -> Send Multipacket UDP/6(transmitId)
  File Logger Wrapper/1(UDP Data) -> Send Multipacket UDP/5(Data)
  sIP/1 -> Send Multipacket UDP/1(sourceIP)
  dIP/1 -> Send Multipacket UDP/2(destIP)
  sPort/1 -> Send Multipacket UDP/3(sourcePort)
  dPort/1 -> Send Multipacket UDP/4(destPort)
  Enable/1 -> Send Multipacket UDP/Enable
  Data/1 -> File Logger Wrapper/3(Frame)
  DataLen/1 -> File Logger Wrapper/4(FrameSize)
  File Logger Wrapper/2(UDP Size) -> ?
  MATLAB Function1/1(y) -> File Logger Wrapper/2(FileName)
  Packet Type/1 -> File Logger Wrapper/1(Packet Type)
  FileName/1 -> MATLAB Function1/1(u)

== system rigLoggerMultipacketRigH/Discrete Data & Format/File Logger Format/File Logger Multipacket ==
  Packet Type : Inport
  FileName : Inport  Port=2
  Data : Inport  Port=3
  DataLen : Inport  Port=4
  transmitID : Inport  Port=5
  Enable : Inport  Port=6
  File Logger Wrapper : Subsystem
  MATLAB Function1 : MATLAB Function  TreatAsAtomicUnit=on
  Send Multipacket UDP : Subsystem  mask(Send Multipacket UDP Block){destMac=macaddr('ff:ff:ff:ff:ff:ff'), ID=2, prependHeader=off}
      mask prompts: destMac "Destination MAC:"; ID "Ethernet Device ID:"; prependHeader "Prepend 4-byte Header (uint16 length, uint16 checksum)"
      mask help: Splits a UDP packet into multiple pieces to be reassembled at the receiver
      mask TypeOptions ID: Ethernet Tx /ID
      mask Display:
      | disp([ 'Ethernet Tx ' num2str(ID)]);
      | port_label('input', 1, 'sourceIp');
      | port_label('input', 2, 'destIp');
      | port_label('input', 3, 'sourcePort');
      | port_label('input', 4, 'destPort');
      | port_label('input', 5, 'data (uint8)');
      | port_label('input', 6, 'transmitId (uint8)');
      | port_label('Enable','Enable')
  dIP : Constant  Value=modelConstants.filelogging.ip  OutDataTypeStr=uint8
  dPort : Constant  Value=modelConstants.filelogging.RECV_PORT  OutDataTypeStr=uint16
  sIP : Constant  Value=modelConstants.filelogging.xPCip  OutDataTypeStr=uint8
  sPort : Constant  Value=modelConstants.filelogging.SRC_PORT  OutDataTypeStr=uint16
  wires:
  transmitID/1 -> Send Multipacket UDP/6(transmitId)
  File Logger Wrapper/1(UDP Data) -> Send Multipacket UDP/5(Data)
  sIP/1 -> Send Multipacket UDP/1(sourceIP)
  dIP/1 -> Send Multipacket UDP/2(destIP)
  sPort/1 -> Send Multipacket UDP/3(sourcePort)
  dPort/1 -> Send Multipacket UDP/4(destPort)
  Enable/1 -> Send Multipacket UDP/Enable
  Data/1 -> File Logger Wrapper/3(Frame)
  DataLen/1 -> File Logger Wrapper/4(FrameSize)
  File Logger Wrapper/2(UDP Size) -> ?
  MATLAB Function1/1(y) -> File Logger Wrapper/2(FileName)
  Packet Type/1 -> File Logger Wrapper/1(Packet Type)
  FileName/1 -> MATLAB Function1/1(u)

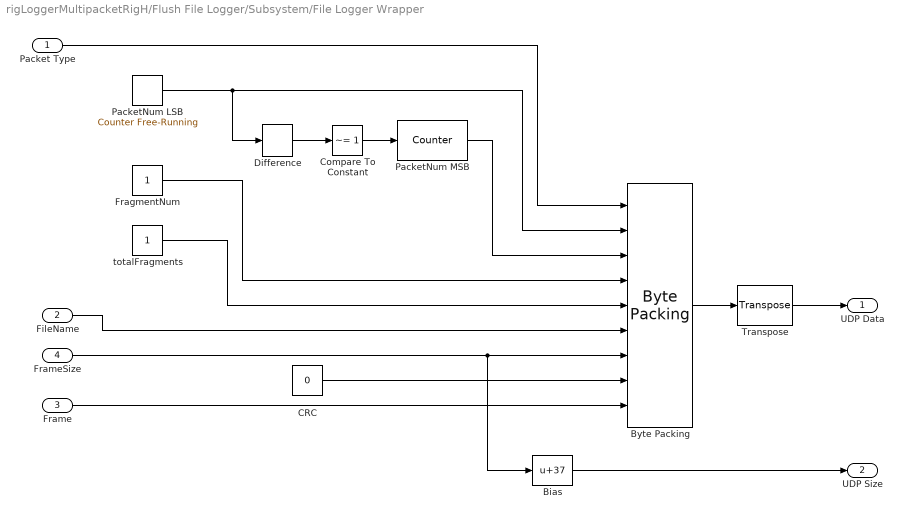
== system rigLoggerMultipacketRigH/Flush File Logger/Subsystem/File Logger Wrapper ==
  Packet Type : Inport
  FileName : Inport  Port=2
  Frame : Inport  Port=3
  FrameSize : Inport  Port=4
  Bias : Bias  Bias=37
  "Byte Packing " : xpcutilitieslib/Byte Packing   MaskPackedDataType=uint8  MaskUnpackedDataTypes={'boolean' 'uint32' 'uint32' 'uint8' 'uint8' 'uint8' 'uint16' 'uint32' 'uint8'}  MaskAlignment=1
  CRC : Constant  Value=0  OutDataTypeStr=uint32
  Compare To Constant : simulink/Logic and Bit Operations/Compare To Constant  relop=~=  const=1  OutDataTypeStr=uint8  ZeroCross=off
  Difference : simulink/Discrete/Difference  ICPrevInput=0  InputProcessing=Inherited  OutMin=[]  OutMax=[]  OutDataType=fixdt(1, 16)  OutScaling=2^-10  DoSatur=off
  FragmentNum : Constant  OutDataTypeStr=uint8
  PacketNum LSB : simulink/Sources/Counter Free-Running  NumBits=32  tsamp=-1
  PacketNum MSB : dspswit3/Counter  Direction=Up  CountEvent=Non-zero sample  CounterSize=32 bits  MaxCount=255  InitialCount=0  Output=Count  HitValue=32  ResetInput=off  SamplesPerFrame=1  Ts=1  CntDtype=uint32  HitDtype=Logical
  Transpose : dspmtrx3/Transpose  Hermitian=off  overflowFlag=off
  totalFragments : Constant  OutDataTypeStr=uint8
  UDP Data : Outport
  UDP Size : Outport  Port=2
  wires:
  Transpose/1 -> UDP Data/1
  "Byte Packing "/1 -> Transpose/1
  Frame/1 -> "Byte Packing "/9
  FrameSize/1 -> Bias/1, "Byte Packing "/7
  CRC/1 -> "Byte Packing "/8
  PacketNum MSB/1 -> "Byte Packing "/3
  Compare To Constant/1 -> PacketNum MSB/1
  Difference/1 -> Compare To Constant/1
  Packet Type/1 -> "Byte Packing "/1
  PacketNum LSB/1 -> "Byte Packing "/2, Difference/1
  FragmentNum/1 -> "Byte Packing "/4
  totalFragments/1 -> "Byte Packing "/5
  FileName/1 -> "Byte Packing "/6
  Bias/1 -> UDP Size/1

== system rigLoggerMultipacketRigH/Flush File Logger/Subsystem/Send Multipacket UDP ==
  sourceIP : Inport
  destIP : Inport  Port=2
  sourcePort : Inport  Port=3
  destPort : Inport  Port=4
  Data : Inport  Port=5  OutDataTypeStr=uint8
  transmitId : Inport  Port=6  OutDataTypeStr=uint8
  Enable : EnablePort
  "Ethernet Tx " : xpcethernetlib/Ethernet Tx   ID=2  SampleTime=-1
  For Iterator Subsystem : Subsystem  TreatAsAtomicUnit=on
  "Link " : xpcnetworkbufferlib/Link 
  MATLAB Function : MATLAB Function  TreatAsAtomicUnit=on
  MATLAB Function1 : MATLAB Function  TreatAsAtomicUnit=on
  TransmitBlockId1 : Constant  Value=uint8(prependHeader)  OutDataTypeStr=uint8
  wires:
  destPort/1 -> For Iterator Subsystem/7(destPort)
  sourcePort/1 -> For Iterator Subsystem/6(sourcePort)
  destIP/1 -> For Iterator Subsystem/5(destIP)
  sourceIP/1 -> For Iterator Subsystem/4(sourceIP)
  MATLAB Function/1(numPackets) -> For Iterator Subsystem/2(Num Packets)
  Data/1 -> MATLAB Function/1(in), For Iterator Subsystem/1(Data)
  transmitId/1 -> MATLAB Function1/1(transmitId)
  MATLAB Function1/1(datagramId) -> For Iterator Subsystem/3(Datagram Id)
  TransmitBlockId1/1 -> MATLAB Function/2(prependHeader)
  For Iterator Subsystem/1(NB Vector) -> "Link "/1
  "Link "/1 -> "Ethernet Tx "/1

== system rigLoggerMultipacketRigH/Neural Data & Format1/File Logger Data/File Logger Multipacket ==
  Packet Type : Inport
  FileName : Inport  Port=2
  Data : Inport  Port=3
  DataLen : Inport  Port=4
  transmitID : Inport  Port=5
  Enable : Inport  Port=6
  File Logger Wrapper : Subsystem
  MATLAB Function1 : MATLAB Function  TreatAsAtomicUnit=on
  Send Multipacket UDP : Subsystem  mask(Send Multipacket UDP Block){destMac=macaddr('ff:ff:ff:ff:ff:ff'), ID=2, prependHeader=off}
      mask prompts: destMac "Destination MAC:"; ID "Ethernet Device ID:"; prependHeader "Prepend 4-byte Header (uint16 length, uint16 checksum)"
      mask help: Splits a UDP packet into multiple pieces to be reassembled at the receiver
      mask TypeOptions ID: Ethernet Tx /ID
      mask Display:
      | disp([ 'Ethernet Tx ' num2str(ID)]);
      | port_label('input', 1, 'sourceIp');
      | port_label('input', 2, 'destIp');
      | port_label('input', 3, 'sourcePort');
      | port_label('input', 4, 'destPort');
      | port_label('input', 5, 'data (uint8)');
      | port_label('input', 6, 'transmitId (uint8)');
      | port_label('Enable','Enable')
  dIP : Constant  Value=modelConstants.filelogging.ip  OutDataTypeStr=uint8
  dPort : Constant  Value=modelConstants.filelogging.RECV_PORT  OutDataTypeStr=uint16
  sIP : Constant  Value=modelConstants.filelogging.xPCip  OutDataTypeStr=uint8
  sPort : Constant  Value=modelConstants.filelogging.SRC_PORT  OutDataTypeStr=uint16
  wires:
  transmitID/1 -> Send Multipacket UDP/6(transmitId)
  File Logger Wrapper/1(UDP Data) -> Send Multipacket UDP/5(Data)
  sIP/1 -> Send Multipacket UDP/1(sourceIP)
  dIP/1 -> Send Multipacket UDP/2(destIP)
  sPort/1 -> Send Multipacket UDP/3(sourcePort)
  dPort/1 -> Send Multipacket UDP/4(destPort)
  Enable/1 -> Send Multipacket UDP/Enable
  Data/1 -> File Logger Wrapper/3(Frame)
  DataLen/1 -> File Logger Wrapper/4(FrameSize)
  File Logger Wrapper/2(UDP Size) -> ?
  MATLAB Function1/1(y) -> File Logger Wrapper/2(FileName)
  Packet Type/1 -> File Logger Wrapper/1(Packet Type)
  FileName/1 -> MATLAB Function1/1(u)

== system rigLoggerMultipacketRigH/Neural Data & Format1/File Logger Format/File Logger Multipacket ==
  Packet Type : Inport
  FileName : Inport  Port=2
  Data : Inport  Port=3
  DataLen : Inport  Port=4
  transmitID : Inport  Port=5
  Enable : Inport  Port=6
  File Logger Wrapper : Subsystem
  MATLAB Function1 : MATLAB Function  TreatAsAtomicUnit=on
  Send Multipacket UDP : Subsystem  mask(Send Multipacket UDP Block){destMac=macaddr('ff:ff:ff:ff:ff:ff'), ID=2, prependHeader=off}
      mask prompts: destMac "Destination MAC:"; ID "Ethernet Device ID:"; prependHeader "Prepend 4-byte Header (uint16 length, uint16 checksum)"
      mask help: Splits a UDP packet into multiple pieces to be reassembled at the receiver
      mask TypeOptions ID: Ethernet Tx /ID
      mask Display:
      | disp([ 'Ethernet Tx ' num2str(ID)]);
      | port_label('input', 1, 'sourceIp');
      | port_label('input', 2, 'destIp');
      | port_label('input', 3, 'sourcePort');
      | port_label('input', 4, 'destPort');
      | port_label('input', 5, 'data (uint8)');
      | port_label('input', 6, 'transmitId (uint8)');
      | port_label('Enable','Enable')
  dIP : Constant  Value=modelConstants.filelogging.ip  OutDataTypeStr=uint8
  dPort : Constant  Value=modelConstants.filelogging.RECV_PORT  OutDataTypeStr=uint16
  sIP : Constant  Value=modelConstants.filelogging.xPCip  OutDataTypeStr=uint8
  sPort : Constant  Value=modelConstants.filelogging.SRC_PORT  OutDataTypeStr=uint16
  wires:
  transmitID/1 -> Send Multipacket UDP/6(transmitId)
  File Logger Wrapper/1(UDP Data) -> Send Multipacket UDP/5(Data)
  sIP/1 -> Send Multipacket UDP/1(sourceIP)
  dIP/1 -> Send Multipacket UDP/2(destIP)
  sPort/1 -> Send Multipacket UDP/3(sourcePort)
  dPort/1 -> Send Multipacket UDP/4(destPort)
  Enable/1 -> Send Multipacket UDP/Enable
  Data/1 -> File Logger Wrapper/3(Frame)
  DataLen/1 -> File Logger Wrapper/4(FrameSize)
  File Logger Wrapper/2(UDP Size) -> ?
  MATLAB Function1/1(y) -> File Logger Wrapper/2(FileName)
  Packet Type/1 -> File Logger Wrapper/1(Packet Type)
  FileName/1 -> MATLAB Function1/1(u)
